simulink model "qn1"  (R2019b)
settings: Solver=ode4  StartTime=0.0  StopTime=10.0  FixedStep=0.001  RelTol=1e-3  EnableMultiTasking=on
libraries: simulink x2
settings Model: Creator=amir  LastModifiedBy=MHTRON001
settings SolverCC: AutoInsertRateTranBlk=on
settings DataIOCC: LimitDataPoints=on  SaveFormat=Array  SignalLoggingSaveFormat=ModelDataLogs  ReturnWorkspaceOutputs=off
settings OptimizationCC: ExpressionDepthLimit=2147483647  LifeSpan=inf
settings DebuggingCC: UnderspecifiedInitializationDetection=Classic  MergeDetectMultiDrivingBlocksExec=none  SolverPrmCheckMsg=warning  FcnCallInpInsideContextMsg=warning  StateNameClashWarn=warning  SFUnexpectedBacktrackingDiag=warning  SFNoUnconditionalDefaultTransitionDiag=warning  SFExecutionAtInitializationDiag=none  ArithmeticOperatorsInVariantConditions=warning
settings HardwareCC: ProdBitPerPointer=32  ProdBitPerSizeT=32  ProdBitPerPtrDiffT=32  ProdLargestAtomicFloat=None  ProdIntDivRoundTo=Undefined  ProdEndianess=Unspecified  ProdWordSize=32  ProdHWDeviceType=32-bit Generic
settings ModelReferenceCC: PropagateSignalLabelsOutOfModel=off
settings SFSimCC: SimUseLocalCustomCode=off  CustomCodeUndefinedFunction=UseInterfaceOnly
settings RTWCC: RTWUseLocalCustomCode=off
settings CodeAppCC: StateflowObjectComments=on
settings GRTTargetCC: TargetLangStandard=C89/C90 (ANSI)  GeneratePreprocessorConditionals=Disable all
settings ConfigComp: CovMetricSettings=dw  CovHtmlReporting=on  CovSaveCumulativeToWorkspaceVar=on  CovSaveSingleToWorkspaceVar=on  CovExternalEMLEnable=off

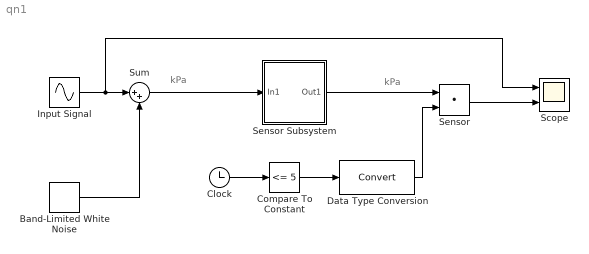
== system qn1 ==
  note: kPa
  note: kPa
  " Input Signal " : Sin  SampleTime=0
  Band-Limited White Noise : simulink/Sources/Band-Limited White Noise  Cov=0.5*0.02  Ts=0.02  seed=[23242]
  Clock : Clock
  Compare To Constant : simulink/Logic and Bit Operations/Compare To Constant  relop=<=  const=5  OutDataTypeStr=boolean
  Data Type Conversion : DataTypeConversion
  Scope : Scope  NumInputPorts=2
  Sensor : DotProduct  InputSameDT=on  OutDataTypeStr=Inherit: Inherit via internal rule
  Sensor Subsystem : Subsystem
  Sum : Sum  Inputs=|++
  wires:
  " Input Signal "/1 -> Scope/1, Sum/1
  Band-Limited White Noise/1 -> Sum/2
  Sum/1 -> Sensor Subsystem/1(In1)
  Sensor Subsystem/1(Out1) -> Sensor/1
  Clock/1 -> Compare To Constant/1
  Compare To Constant/1 -> Data Type Conversion/1
  Data Type Conversion/1 -> Sensor/2
  Sensor/1 -> Scope/2

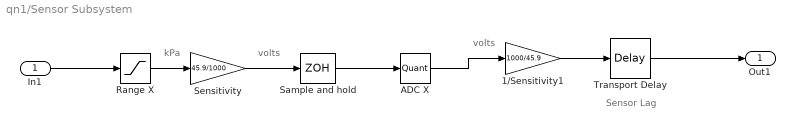
== system qn1/Sensor Subsystem ==
  note: kPa
  note: volts
  note: volts
  note: Sensor Lag
  In1 : Inport
  1/Sensitivity1 : Gain  Gain=1000/45.9
  ADC X : Quantizer  QuantizationInterval=5/65536
  Range X : Saturate  UpperLimit=115  LowerLimit=-15
  Sample and hold : ZeroOrderHold  SampleTime=0.02
  Sensitivity : Gain  Gain=45.9/1000
  Transport Delay : TransportDelay  DelayTime=0.5
  Out1 : Outport
  wires:
  Sample and hold/1 -> ADC X/1
  1/Sensitivity1/1 -> Transport Delay/1
  Sensitivity/1 -> Sample and hold/1
  ADC X/1 -> 1/Sensitivity1/1
  Transport Delay/1 -> Out1/1
  Range X/1 -> Sensitivity/1
  In1/1 -> Range X/1
